simulink model "goodwin_comparacion"  (R2024b)
settings: Solver=VariableStepAuto  StartTime=0.0  StopTime=tmax  MaxStep=1e-3
undefined symbols (not defined in the file or in its folder): A, alpha, B, beta, C, D, delta, nu, phi0, phi1, x0, x10, x20
settings DataIOCC: ReturnWorkspaceOutputs=off

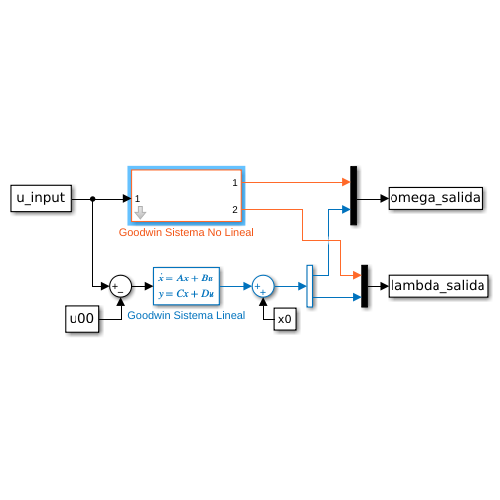
[thumbnail: Simulink's stored preview of the top-level diagram]
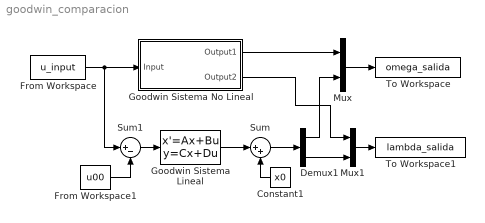
== system goodwin_comparacion ==
  Constant1 : Constant  Value=x0
  Demux1 : Demux  Outputs=2
  From Workspace : FromWorkspace  VariableName=u_input
  From Workspace1 : FromWorkspace  VariableName=u00
  Goodwin Sistema Lineal : StateSpace  A=A  B=B  C=C  D=D  InitialCondition=0
  Goodwin Sistema No Lineal : Subsystem  mask(Modelo Goodwin){nu=nu, alpha=alpha, beta=beta, phi0=phi0, phi1=phi1, x0=[x10 x20]}
      mask prompts: x0 "c.i"
      mask help:
      | nu (ν): Tasa de capital a salida.
      | alpha (α): Tasa de crecimiento de la productividad.
      | beta (β): Tasa de crecimiento de la población.
      | delta (δ): Tasa de depreciación del capital.
      | phi1 (φ1) y phi0 (φ0): Parámetros de la curva de Phillips.
      mask Help:
      | Ecuaciones del modelo:
      | 
      | La tasa de cambio de x1 (proporción salarial) está dada por:
      | 
      | dx1/dt = x1 * [(phi1 / (1 - x2)^2) - phi0 - alpha]
      | Esto significa que la proporción salarial cambia en función del valor actual de la proporción salarial, el parámetro phi1, la tasa de empleo x2, el parámetro base phi0, y la tasa de crecimiento de la productividad alpha.
      | 
      | La tasa de cambio de x2 (tasa de empleo) está dada por:
      | 
      | dx2/dt = x2 * [(1 - x1) / nu - alpha - beta - delta] + u_input
      | Esto indica que la tasa de empleo cambia en función de su valor actual, la proporción salarial x1, el parámetro nu, la tasa de crecimiento de la productividad alpha, la tasa de crecimiento de la población beta, la tasa de depreciación del capital delta, y un factor externo representado por u_input.
      | 
      | La ecuación para la producción económica está dada por:
      | 
      | Y_output(t) = Y0 * (x2(t) / x2(0)) * exp((alpha + beta) * t)
      | Esto significa que la producción económica en el tiempo t depende del valor inicial de la producción Y0, la tasa de empleo en el tiempo t, la tasa de empleo inicial x2(0), y la combinación de las tasas de crecimiento de la productividad alpha y de la población beta.
  Mux : Mux  Inputs=2
  Mux1 : Mux  Inputs=2
  Sum : Sum  Inputs=|++
  Sum1 : Sum  Inputs=|+-
  To Workspace : ToWorkspace  VariableName=omega_salida  SaveFormat=Structure With Time  SampleTime=-1
  To Workspace1 : ToWorkspace  VariableName=lambda_salida  SaveFormat=Structure With Time  SampleTime=-1
  wires:
  From Workspace/1 -> Sum1/1, Goodwin Sistema No Lineal/1(Input)
  Goodwin Sistema No Lineal/1(Output1) -> Mux/1
  Goodwin Sistema Lineal/1 -> Sum/1
  Sum/1 -> Demux1/1
  Sum1/1 -> Goodwin Sistema Lineal/1
  Mux1/1 -> To Workspace1/1
  From Workspace1/1 -> Sum1/2
  Constant1/1 -> Sum/2
  Mux/1 -> To Workspace/1
  Goodwin Sistema No Lineal/2(Output2) -> Mux1/1
  Demux1/1 -> Mux/2
  Demux1/2 -> Mux1/2

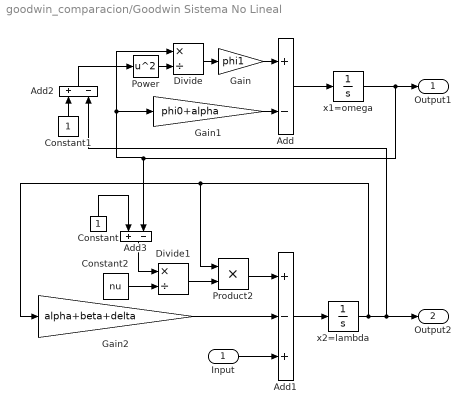
== system goodwin_comparacion/Goodwin Sistema No Lineal ==
  Input : Inport
  Add : Sum  Inputs=+-
  Add1 : Sum  Inputs=+-+
  Add2 : Sum  Inputs=+-
  Add3 : Sum  Inputs=+-
  Constant : Constant
  Constant1 : Constant
  Constant2 : Constant  Value=nu
  Divide : Product  Inputs=*/
  Divide1 : Product  Inputs=*/
  Gain : Gain  Gain=phi1
  Gain1 : Gain  Gain=phi0+alpha
  Gain2 : Gain  Gain=alpha+beta+delta
  Power : Math  Operator=square
  Product2 : Product
  x1=omega : Integrator  InitialCondition=x10
  x2=lambda : Integrator  InitialCondition=x20
  Output1 : Outport
  Output2 : Outport  Port=2
  wires:
  Gain2/1 -> Add1/2
  Constant1/1 -> Add2/1
  Add/1 -> x1=omega/1
  x1=omega/1 -> Gain1/1, Divide/1, Add3/2, Output1/1
  Gain1/1 -> Add/2
  Add3/1 -> Divide1/1
  Add1/1 -> x2=lambda/1
  x2=lambda/1 -> Output2/1, Add2/2, Gain2/1, Product2/1
  Constant/1 -> Add3/1
  Power/1 -> Divide/2
  Gain/1 -> Add/1
  Divide/1 -> Gain/1
  Constant2/1 -> Divide1/2
  Add2/1 -> Power/1
  Input/1 -> Add1/3
  Divide1/1 -> Product2/2
  Product2/1 -> Add1/1
